simulink model "MBD_problem_1"  (R2020b)
settings: Solver=VariableStepAuto  StartTime=0.0  StopTime=10.0  RelTol=1e-3
InitFcn:
  | M1=100;
  | k1=50;
  | b=50;
  | k12=500;
  | M2=5;
settings Model: Creator=Lenovo  LastModifiedBy=Lenovo

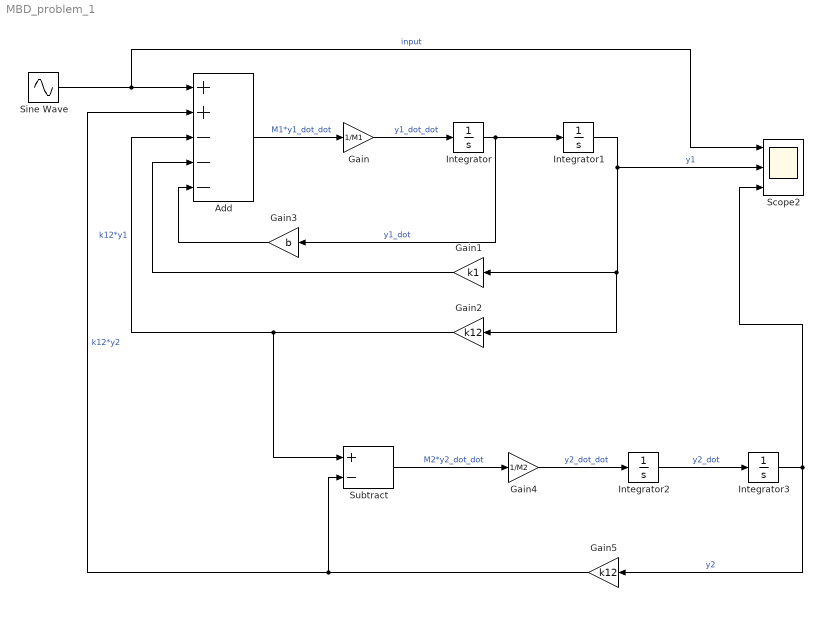
== system MBD_problem_1 ==
  Add : Sum  Inputs=++---
  Gain : Gain  Gain=1/M1
  Gain1 : Gain  Gain=k1
  Gain2 : Gain  Gain=k12
  Gain3 : Gain  Gain=b
  Gain4 : Gain  Gain=1/M2
  Gain5 : Gain  Gain=k12
  Integrator{,1..3} (4 alike) : Integrator
  Scope2 : Scope  NumInputPorts=3
  Sine Wave : Sin  Amplitude=2  Frequency=1.59  SampleTime=0
  Subtract : Sum  Inputs=+-
  wires:
  Add/1 -> Gain/1  "M1*y1_dot_dot"
  Gain2/1 -> Subtract/1, Add/3  "k12*y1"
  Gain3/1 -> Add/5
  Integrator2/1 -> Integrator3/1  "y2_dot"
  Sine Wave/1 -> Scope2/1, Add/1  "input"
  Gain1/1 -> Add/4
  Integrator3/1 -> Scope2/3, Gain5/1  "y2"
  Gain/1 -> Integrator/1  "y1_dot_dot"
  Gain4/1 -> Integrator2/1  "y2_dot_dot"
  Subtract/1 -> Gain4/1  "M2*y2_dot_dot"
  Gain5/1 -> Add/2, Subtract/2  "k12*y2"
  Integrator/1 -> Gain3/1, Integrator1/1  "y1_dot"
  Integrator1/1 -> Gain2/1, Gain1/1, Scope2/2  "y1"
